simulink model "W04_3_heading_offline"  (R2024b)
settings: Solver=ode4  StartTime=0.0  StopTime=40  FixedStep=0.05  RelTol=1e-3
values from neighbouring files (symbols this model uses):
  animate = 1    [W04_setup.m]
  head_open = 0    [W04_setup.m]
  Kd_psi = 400    [W04_setup.m]
  Ki_psi = 0    [W04_setup.m]
  Kp_psi = 800    [W04_setup.m]
  N_max = 500    [W04_setup.m]
  N_open = 300    [W04_setup.m]
  port_eff = 1.0    (= 1)    [W04_setup.m]
  psi_ref_deg = 45    [W04_setup.m]
  settle_band = 1.0    (= 1)    [W04_setup.m]
  settle_hold = 5.0    (= 5)    [W04_setup.m]
  use_ssa = 1    [W04_setup.m]
  X_head = 300    [W04_setup.m]
settings Model: Creator=admin  LastModifiedBy=admin

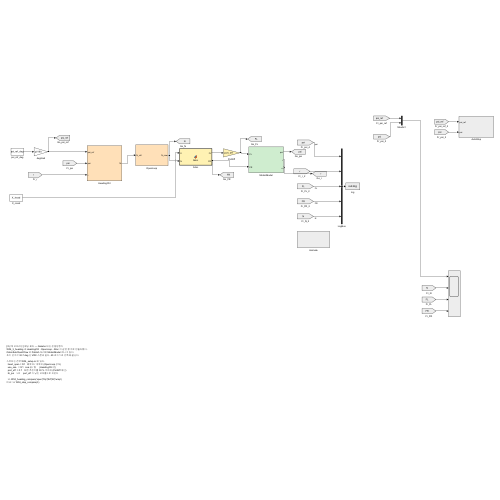
[thumbnail: Simulink's stored preview of the top-level diagram]
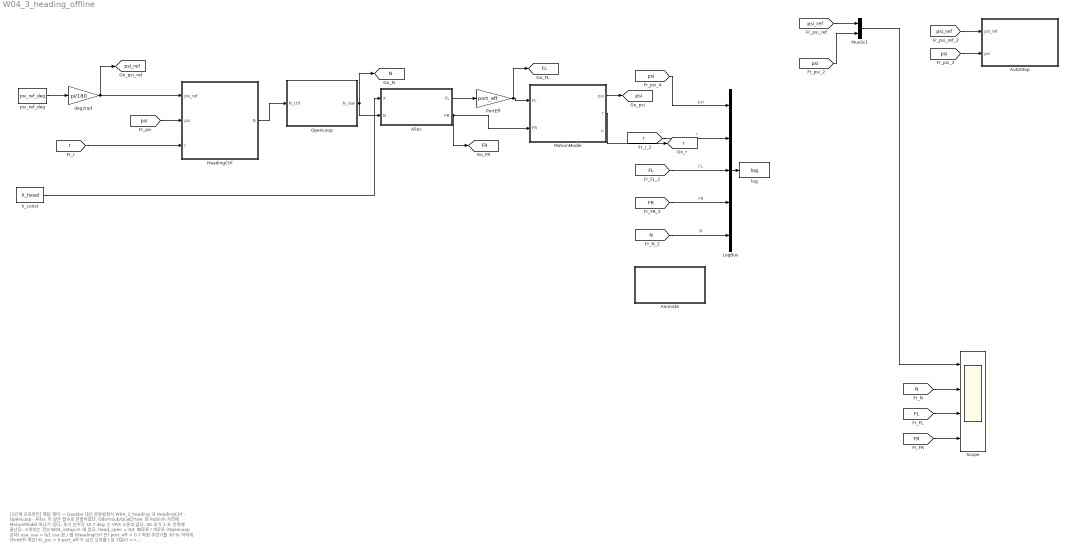
== system W04_3_heading_offline ==
  note: [3단계 오프라인] 헤딩 제어 — Gazebo 대신 운동방정식
      | W04_3_heading 과 HeadingCtrl · OpenLoop · Alloc 이 같은 함수로 만들어졌다.
      | OdomSub/Quat2Yaw 와 Publish 자리에 MotionModel 하나가 있다.
      | 초기 선수각 32.7 deg 는 VRX 스폰과 같다. 40 초가 1 초 안쪽에 끝난다.
      |
      | 스위치는 전부 W04_setup.m 에 있다.
      |   head_open = 0/1   폐루프 / 개루프 (OpenLoop 상자)
      |   use_ssa   = 0/1   ssa 끔 / 켬     (HeadingCtrl 안)
      |   port_eff  = 0.7   좌현 추진기를 30 % 약하게 (PortEff 게인)
      |   Ki_psi    > 0     port_eff 가 남긴 오차를 I 로 지운다
      |
      |   >> W04_heading_compare('open'|'Kp'|'Kd'|'Ki'|'wrap')
      | 비교: >> W04_step_compare(3)
  Alloc : MATLAB Function  TreatAsAtomicUnit=on
  Animate : Subsystem
  AutoStop : Subsystem
  HeadingCtrl : Subsystem
  LogBus : BusCreator  Inputs=5
  MotionModel : Subsystem
  MuxSc1 : Mux  Inputs=2
  OpenLoop : Subsystem
  PortEff : Gain  Gain=port_eff
  Scope : Scope  NumInputPorts=4
  X_const : Constant  Value=X_head
  deg2rad : Gain  Gain=pi/180
  log : ToWorkspace  VariableName=log  SaveFormat=Timeseries  SampleTime=0.05
  psi_ref_deg : Constant  Value=psi_ref_deg
  tag scope: FL=global, FR=global, N=global, psi=global, psi_ref=global, r=global
  wires:
  X_const/1 -> Alloc/1(X)
  HeadingCtrl/1(N) -> OpenLoop/1(N_ctrl)
  psi_ref_deg/1 -> deg2rad/1
  deg2rad/1 -> HeadingCtrl/1(psi_ref), [psi_ref]
  [psi] -> HeadingCtrl/2(psi)
  [r] -> HeadingCtrl/3(r)
  Alloc/1(FL) -> PortEff/1
  PortEff/1 -> MotionModel/1(FL), [FL]
  Alloc/2(FR) -> MotionModel/2(FR), [FR]
  MotionModel/1(psi) -> [psi]
  [psi_ref] -> MuxSc1/1
  [psi] -> MuxSc1/2
  [psi_ref] -> AutoStop/1(psi_ref)
  [psi] -> AutoStop/2(psi)
  [psi] -> LogBus/1  "psi"
  [FL] -> LogBus/3  "FL"
  [FR] -> LogBus/4  "FR"
  [N] -> LogBus/5  "N"
  LogBus/1 -> log/1
  MuxSc1/1 -> Scope/1
  [FL] -> Scope/3
  [FR] -> Scope/4
  [N] -> Scope/2
  OpenLoop/1(N_raw) -> Alloc/2(N), [N]
  MotionModel/2(r) -> [r]
  [r] -> LogBus/2  "r"

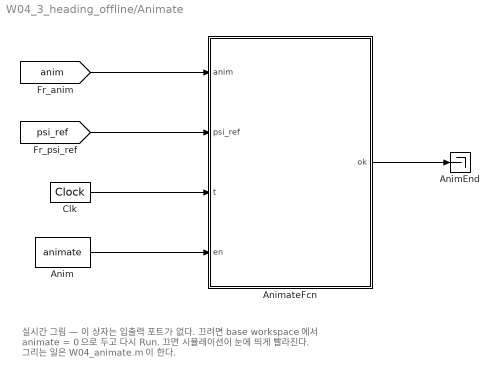
== system W04_3_heading_offline/Animate ==
  note: 실시간 그림 — 이 상자는 입출력 포트가 없다.
      | 끄려면 base workspace 에서  animate = 0  으로 두고 다시 Run.
      | 끄면 시뮬레이션이 눈에 띄게 빨라진다.
      | 그리는 일은 W04_animate.m 이 한다.
  Anim : Constant  Value=animate
  AnimEnd : Terminator
  AnimateFcn : MATLAB Function  TreatAsAtomicUnit=on
  Clk : DigitalClock  SampleTime=0.05
  wires:
  [anim] -> AnimateFcn/1(anim)
  [psi_ref] -> AnimateFcn/2(psi_ref)
  Clk/1 -> AnimateFcn/3(t)
  Anim/1 -> AnimateFcn/4(en)
  AnimateFcn/1(ok) -> AnimEnd/1

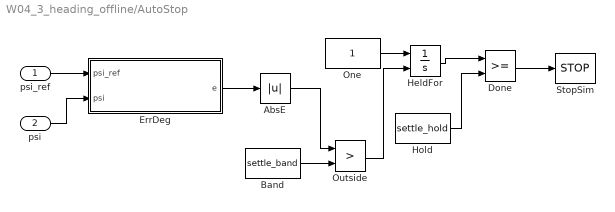
== system W04_3_heading_offline/AutoStop ==
  psi_ref : Inport
  psi : Inport  Port=2
  AbsE : Abs  SaturateOnIntegerOverflow=off
  Band : Constant  Value=settle_band
  Done : RelationalOperator  OutDataTypeStr=boolean  RndMeth=Simplest  InputSameDT=off
  ErrDeg : MATLAB Function  TreatAsAtomicUnit=on
  HeldFor : Integrator  ExternalReset=level
  Hold : Constant  Value=settle_hold
  One : Constant
  Outside : RelationalOperator  Operator=>  OutDataTypeStr=boolean  RndMeth=Simplest  InputSameDT=off
  StopSim : Stop
  wires:
  psi_ref/1 -> ErrDeg/1(psi_ref)
  psi/1 -> ErrDeg/2(psi)
  AbsE/1 -> Outside/1
  Outside/1 -> HeldFor/2
  ErrDeg/1(e) -> AbsE/1
  HeldFor/1 -> Done/1
  Band/1 -> Outside/2
  Hold/1 -> Done/2
  One/1 -> HeldFor/1
  Done/1 -> StopSim/1

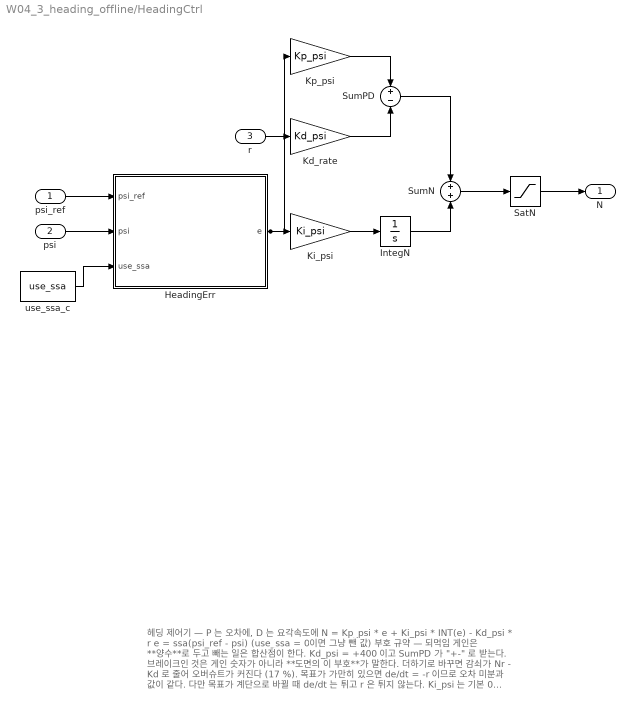
== system W04_3_heading_offline/HeadingCtrl ==
  note: 헤딩 제어기 — P 는 오차에, D 는 요각속도에
      |
      |     N = Kp_psi * e  +  Ki_psi * INT(e)  -  Kd_psi * r
      |     e = ssa(psi_ref - psi)   (use_ssa = 0 이면 그냥 뺀 값)
      |
      | 부호 규약 — 되먹임 게인은 **양수**로 두고 빼는 일은 합산점이 한다.
      | Kd_psi = +400 이고 SumPD 가 "+-" 로 받는다. 브레이크인 것은 게인
      | 숫자가 아니라 **도면의 이 부호**가 말한다.
      | 더하기로 바꾸면 감쇠가 Nr - Kd 로 줄어 오버슈트가 커진다 (17 %).
      |
      | 목표가 가만히 있으면 de/dt = -r 이므로 오차 미분과 값이 같다.
      | 다만 목표가 계단으로 바뀔 때 de/dt 는 튀고 r 은 튀지 않는다.
      |
      | Ki_psi 는 기본 0 이다. 한쪽 추진기가 약할 때(port_eff < 1)
      | PD 가 남기는 정상상태 오차를 없애는 자리다 (2-10 절 실습에서 켠다).
      | IntegN 은 **연속** 적분기이고 +-N_max 포화가 걸려 있다
      | (clamping 안티와인드업). 모델 솔버는 고정스텝 ode4 다.
      |
      | SatN 의 +-N_max = 500 N m 는 임의의 수가 아니다. 추진기만으로 낼 수
      | 있는 물리 한계가 2*b_half*F_max = 2*1.027135*250 = 513.57 N m 이고,
      | 500 은 그 97.4 % 다. 전진 추력 X 를 함께 쓰면 2*b_half*(F_max - X/2)
      | 로 줄어, X_head = 300 N 에서는 205.4 N m 가 진짜 한계다 (2-5 절 유도 5).
      |
      | 값은 전부 W04_setup.m — Kp_psi = 800, Kd_psi = +400.
      | 근거는 4주차 극배치 절과 W04_pole_place.m.
  psi_ref : Inport
  psi : Inport  Port=2
  r : Inport  Port=3
  HeadingErr : MATLAB Function  TreatAsAtomicUnit=on
  IntegN : Integrator  LimitOutput=on  UpperSaturationLimit=N_max  LowerSaturationLimit=-N_max
  Kd_rate : Gain  Gain=Kd_psi
  Ki_psi : Gain  Gain=Ki_psi
  Kp_psi : Gain  Gain=Kp_psi
  SatN : Saturate  UpperLimit=N_max  LowerLimit=-N_max
  SumN : Sum
  SumPD : Sum  Inputs=+-
  use_ssa_c : Constant  Value=use_ssa
  N : Outport
  wires:
  psi_ref/1 -> HeadingErr/1(psi_ref)
  psi/1 -> HeadingErr/2(psi)
  use_ssa_c/1 -> HeadingErr/3(use_ssa)
  r/1 -> Kd_rate/1
  Kd_rate/1 -> SumPD/2
  HeadingErr/1(e) -> Kp_psi/1, Ki_psi/1
  Kp_psi/1 -> SumPD/1
  Ki_psi/1 -> IntegN/1
  SumPD/1 -> SumN/1
  IntegN/1 -> SumN/2
  SumN/1 -> SatN/1
  SatN/1 -> N/1

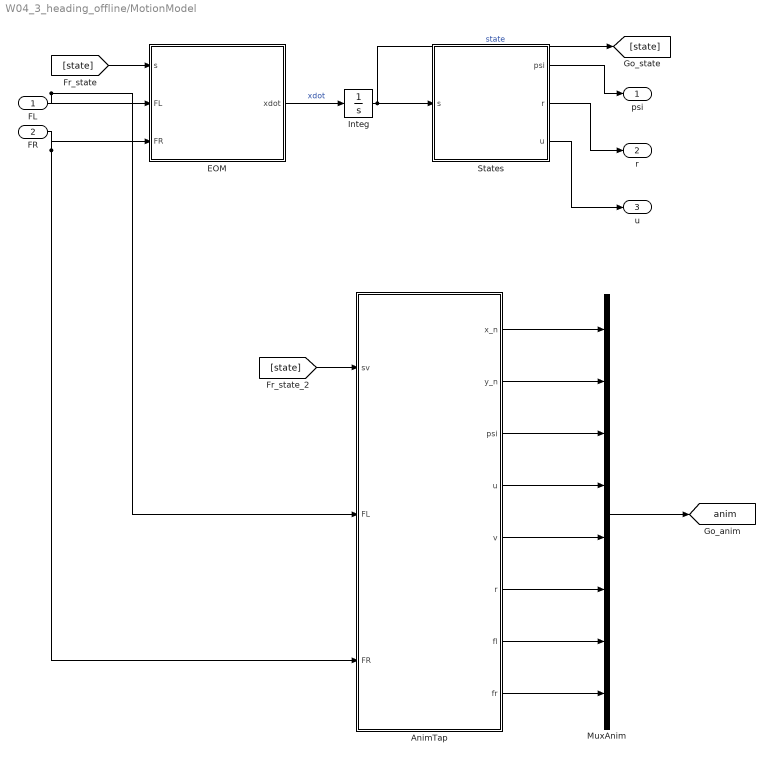
== system W04_3_heading_offline/MotionModel ==
  FL : Inport
  FR : Inport  Port=2
  AnimTap : MATLAB Function  TreatAsAtomicUnit=on
  EOM : MATLAB Function  TreatAsAtomicUnit=on
  Integ : Integrator  InitialCondition=[0;0;0;0;0;32.7*pi/180]
  MuxAnim : Mux  Inputs=8
  States : MATLAB Function  TreatAsAtomicUnit=on
  psi : Outport
  r : Outport  Port=2
  u : Outport  Port=3
  tag scope: anim=global
  wires:
  FL/1 -> EOM/2(FL), AnimTap/2(FL)
  FR/1 -> EOM/3(FR), AnimTap/3(FR)
  EOM/1(xdot) -> Integ/1  "xdot"
  Integ/1 -> States/1(s), [state]  "state"
  States/1(psi) -> psi/1
  States/2(r) -> r/1
  States/3(u) -> u/1
  AnimTap/1(x_n) -> MuxAnim/1
  AnimTap/2(y_n) -> MuxAnim/2
  AnimTap/3(psi) -> MuxAnim/3
  AnimTap/4(u) -> MuxAnim/4
  AnimTap/5(v) -> MuxAnim/5
  AnimTap/6(r) -> MuxAnim/6
  AnimTap/7(fl) -> MuxAnim/7
  AnimTap/8(fr) -> MuxAnim/8
  MuxAnim/1 -> [anim]
  [state] -> EOM/1(s)
  [state] -> AnimTap/1(sv)

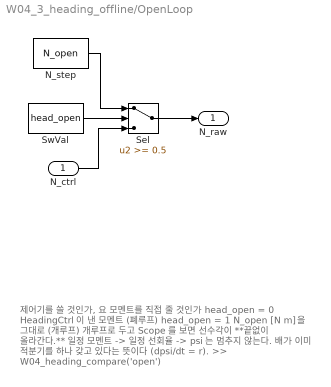
== system W04_3_heading_offline/OpenLoop ==
  note: 제어기를 쓸 것인가, 요 모멘트를 직접 줄 것인가
      |
      |   head_open = 0   HeadingCtrl 이 낸 모멘트 (폐루프)
      |   head_open = 1   N_open [N m] 을 그대로 (개루프)
      |
      | 개루프로 두고 Scope 를 보면 선수각이 **끝없이 올라간다.**
      | 일정 모멘트 -> 일정 선회율 -> psi 는 멈추지 않는다.
      | 배가 이미 적분기를 하나 갖고 있다는 뜻이다 (dpsi/dt = r).
      |
      |   >> W04_heading_compare('open')
  N_ctrl : Inport
  N_step : Constant  Value=N_open
  Sel : Switch  Threshold=0.5  SaturateOnIntegerOverflow=off  InputSameDT=off
  SwVal : Constant  Value=head_open
  N_raw : Outport
  wires:
  N_ctrl/1 -> Sel/3
  N_step/1 -> Sel/1
  SwVal/1 -> Sel/2
  Sel/1 -> N_raw/1

== matlab function W04_3_heading_offline/MotionModel/States ==
  data: s input; psi output; r output; u output
function [psi, r, u] = States(s)
%#codegen
% Quat2Yaw 와 같은 출력 — 선수각은 [-pi, pi] 로 접는다
psi = atan2(sin(s(6)), cos(s(6)));
r = s(3);
u = s(1);

== matlab function W04_3_heading_offline/MotionModel/EOM ==
  data: s input; xdot output; FL input; FR input
function xdot = EOM(s, FL, FR)
%#codegen
% 3-DOF WAM-V equations of motion, NED (3주차 1-8 절).
%   s = [u v r x_n y_n psi]'
m = 211;  Izz = 653;  Xu = 100;  Xuu = 150;  Yv = 100;  Yvv = 100;
Nr = 800;  Nrr = 800;  b_half = 1.027135;
u = s(1); v = s(2); r = s(3); psi = s(6);
X = FL + FR;
N = (FL - FR)*b_half;
du = (X - (Xu + Xuu*abs(u))*u)/m + v*r;
dv = (  - (Yv + Yvv*abs(v))*v)/m - u*r;
dr = (N - (Nr + Nrr*abs(r))*r)/Izz;
xdot = [du; dv; dr;
        u*cos(psi) - v*sin(psi);
        u*sin(psi) + v*cos(psi);
        r];

== matlab function W04_3_heading_offline/MotionModel/AnimTap ==
  data: sv input; x_n output; FL input; FR input; y_n output; psi output; u output; v output; r output; fl output; fr output
function [x_n, y_n, psi, u, v, r, fl, fr] = AnimTap(sv, FL, FR)
%#codegen
% Display-only tap. sv = [u v r x_n y_n psi]'
x_n = sv(4);
y_n = sv(5);
psi = atan2(sin(sv(6)), cos(sv(6)));   % wrap to [-pi, pi]
u   = sv(1);
v   = sv(2);
r   = sv(3);
fl  = FL;
fr  = FR;

== matlab function W04_3_heading_offline/HeadingCtrl/HeadingErr ==
  data: psi_ref input; e output; psi input; use_ssa input
function e = HeadingErr(psi_ref, psi, use_ssa)
%#codegen
% Heading error [rad].
d = psi_ref - psi;
if use_ssa >= 0.5
    % ssa : shortest signed angle, wrapped to (-pi, pi]
    e = atan2(sin(d), cos(d));
else
    % no wrap : 170 deg -> -170 deg becomes -340 deg, not +20 deg
    e = d;
end

== matlab function W04_3_heading_offline/Alloc ==
  data: X input; FL output; N input; FR output
function [FL, FR] = Alloc(X, N)
%#codegen
% Differential thrust allocation for the 2-thruster WAM-V
%   X : surge force  [N]
%   N : yaw moment   [N*m], positive turns to starboard
B_half = 1.027135;      % half distance between thrusters [m]
Fmax   = 250;           % thrust limit per thruster [N]
FL = X/2 + N/(2*B_half);
FR = X/2 - N/(2*B_half);
FL = max(min(FL, Fmax), -Fmax);
FR = max(min(FR, Fmax), -Fmax);

== matlab function W04_3_heading_offline/AutoStop/ErrDeg ==
  data: psi_ref input; e output; psi input
function e = ErrDeg(psi_ref, psi)
%#codegen
% 선수각 오차 [deg], ssa 로 접은 최단 각
d = psi_ref - psi;
e = atan2(sin(d), cos(d)) * 180/pi;

== matlab function W04_3_heading_offline/Animate/AnimateFcn ==
  data: anim input; ok output; psi_ref input; t input; en input
function ok = AnimateFcn(anim, psi_ref, t, en)
%#codegen
% 실시간 그림. MATLAB Function 블록은 그림을 그리지 못하므로 그리는 함수를
% extrinsic 으로 선언한다 — 코드를 만들지 않고 평범한 MATLAB 을 부른다.
% en = base workspace 의 animate (0 이면 그리지 않는다).
%
% anim 은 Mux 로 묶어 온 여덟 신호다 (빌더의 animBundle 과 같은 순서).
%   1 x_n   2 y_n   3 psi   4 u   5 v   6 r   7 FL   8 FR
coder.extrinsic('W04_animate');
ok = 1;
if en > 0.5
    W04_animate(anim(1), anim(2), anim(3), anim(4), anim(5), anim(6), anim(7), anim(8), NaN, psi_ref, t);
end
